simulink model "Controle_Lab4_model"  (R2012b)
settings: Solver=ode45  StartTime=0.0  StopTime=8  RelTol=1e-3
values from neighbouring files (symbols this model uses):
  K = 0.02    [Controle_Lab4.m]    (also in Lab8.m = place(A,B,[-10 -12 -2]); Tarefa1.m)
  Kp = Kkp/K    (= 358.333333333)    [Controle_Lab4.m]    (also in Tarefa1.m = 300)
  KpInt = 0.9 * (T/L)    (= 6.45)    [Controle_Lab4.m]
  L = 1.024 - Start    (= 0.024)    [Controle_Lab4.m]    (also in Tarefa1.m = 0.03)
  T = 1.196 - L - Start    (= 0.172)    [Controle_Lab4.m]    (also in Tarefa1.m = 0.18)
  Ti = L/0.3    (= 0.08)    [Controle_Lab4.m]
settings Model: Creator=11104980  LastModifiedBy=11104980

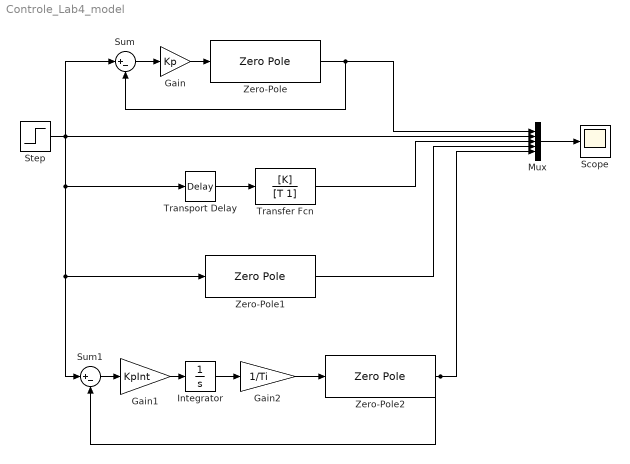
== system Controle_Lab4_model ==
  Gain : Gain  Gain=Kp
  Gain1 : Gain  Gain=KpInt
  Gain2 : Gain  Gain=1/Ti
  Integrator : Integrator
  Mux : Mux  Inputs=5
  Scope : Scope
      settings: SaveName=y
  Step : Step  SampleTime=0
  Sum : Sum  Inputs=|+-
  Sum1 : Sum  Inputs=|+-
  Transfer Fcn : TransferFcn  Numerator=[K]  Denominator=[T 1]
  Transport Delay : TransportDelay  DelayTime=L
  Zero-Pole : ZeroPole  Zeros=[]  Poles=[-20 -25 -30]  Gain=[300]
  Zero-Pole1 : ZeroPole  Zeros=[]  Poles=[-20 -25 -30]  Gain=[300]
  Zero-Pole2 : ZeroPole  Zeros=[]  Poles=[-20 -25 -30]  Gain=[300]
  wires:
  Zero-Pole/1 -> Sum/2, Mux/1
  Mux/1 -> Scope/1
  Transport Delay/1 -> Transfer Fcn/1
  Transfer Fcn/1 -> Mux/3
  Sum/1 -> Gain/1
  Gain/1 -> Zero-Pole/1
  Zero-Pole1/1 -> Mux/4
  Step/1 -> Sum1/1, Zero-Pole1/1, Transport Delay/1, Sum/1, Mux/2
  Zero-Pole2/1 -> Sum1/2, Mux/5
  Sum1/1 -> Gain1/1
  Gain1/1 -> Integrator/1
  Integrator/1 -> Gain2/1
  Gain2/1 -> Zero-Pole2/1
